simulink model "SEIR_simulink"  (R2020b)
settings: Solver=VariableStepAuto  StartTime=0.0  StopTime=300  MaxStep=0.01  RelTol=1e-3
values from neighbouring files (symbols this model uses):
  a = x(1)    [autofitness_fun.m]    (also in fitness_fun.m; fitness_funSEIR.m; provaODE45.m = 1.8; simulationSEIR.m = 1.4)
  b = []    [I_GA.m]    (also in SIR_GA.m; autoSEIR_GA.m; autoSIR_GA.m; autofitness_fun.m = x(2))
  c = n-1    [SIR_GA.m]    (also in autoSEIR_GA.m; autoSIR_GA.m; fitness_funSEIR.m = x(3); simulationSEIR.m = 0.61)
  I0 = I(1)    [I_GA.m]    (also in provaODE45.m = y0(2); simulationSEIR.m = 700)
  N = 60e6    (= 60000000)    [SIR_GA.m]    (also in autoSEIR_GA.m = 59999771; autoSIR_GA.m = 59999771; provaODE45.m = 10000; simulationSEIR.m = 600000)
settings Model: Creator=abd99  LastModifiedBy=abd99

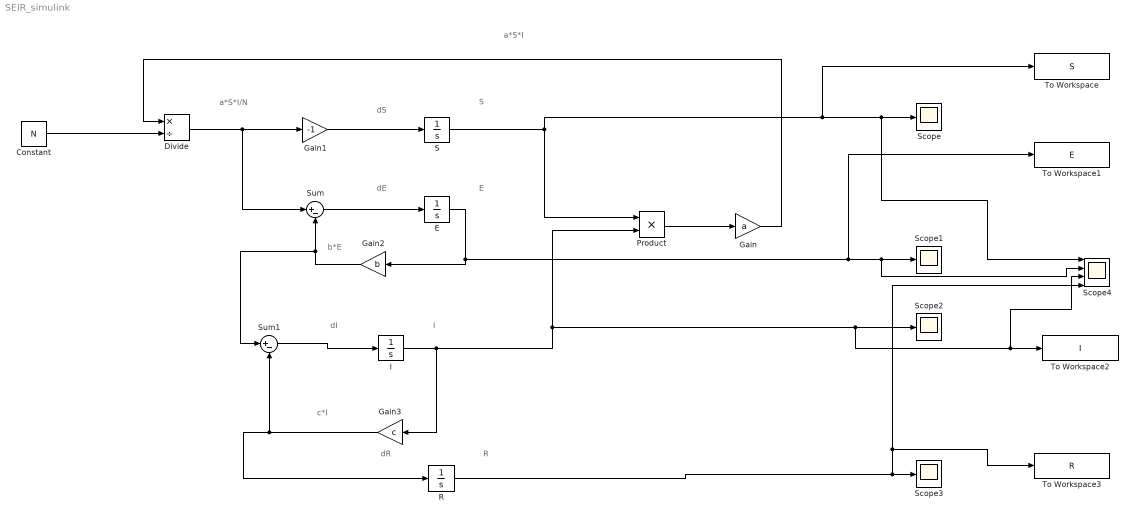
== system SEIR_simulink ==
  note: a*S*I
  note: S
  note: I
  note: dI
  note: E
  note: dE
  note: R
  note: dR
  note: b*E
  note: c*I
  note: dS
  note: a*S*I/N
  Constant : Constant  Value=N
  Divide : Product  Inputs=*/
  E : Integrator
  Gain : Gain  Gain=a
  Gain1 : Gain  Gain=-1
  Gain2 : Gain  Gain=b
  Gain3 : Gain  Gain=c
  I : Integrator  InitialCondition=I0
  Product : Product
  R : Integrator
  S : Integrator  InitialCondition=N
  Scope{,1..3} (4 alike) : Scope
  Scope4 : Scope  NumInputPorts=4
  Sum : Sum  Inputs=|+-
  Sum1 : Sum  Inputs=|+-
  To Workspace : ToWorkspace  VariableName=S  SampleTime=-1
  To Workspace1 : ToWorkspace  VariableName=E  SampleTime=-1
  To Workspace2 : ToWorkspace  VariableName=I  SampleTime=-1
  To Workspace3 : ToWorkspace  VariableName=R  SampleTime=-1
  wires:
  I/1 -> Gain3/1, Scope4/3, To Workspace2/1, Scope2/1, Product/2
  Product/1 -> Gain/1
  Sum/1 -> E/1
  E/1 -> Gain2/1, To Workspace1/1, Scope4/2, Scope1/1
  Gain2/1 -> Sum1/1, Sum/2
  Sum1/1 -> I/1
  Gain3/1 -> R/1, Sum1/2
  R/1 -> To Workspace3/1, Scope4/4, Scope3/1
  Gain1/1 -> S/1
  S/1 -> Product/1, To Workspace/1, Scope4/1, Scope/1
  Divide/1 -> Sum/1, Gain1/1
  Gain/1 -> Divide/1
  Constant/1 -> Divide/2
